simulink library "multiSpoolingController_ul"  (R2020a)
settings: Solver=VariableStepAuto  StartTime=0.0  StopTime=10.0  RelTol=1e-3
undefined symbols (not defined in the file or in its folder): pathCtrl
libraries: firstOrderFilter_ul x1
settings Model: Creator=James Reed  LastModifiedBy=Josh Gaming
settings DataIOCC: ReturnWorkspaceOutputs=off
settings DebuggingCC: ArithmeticOperatorsInVariantConditions=warning
settings SFSimCC: CustomCodeUndefinedFunction=UseInterfaceOnly

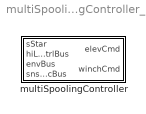
== system multiSpoolingController_ul ==
  multiSpoolingController : Subsystem

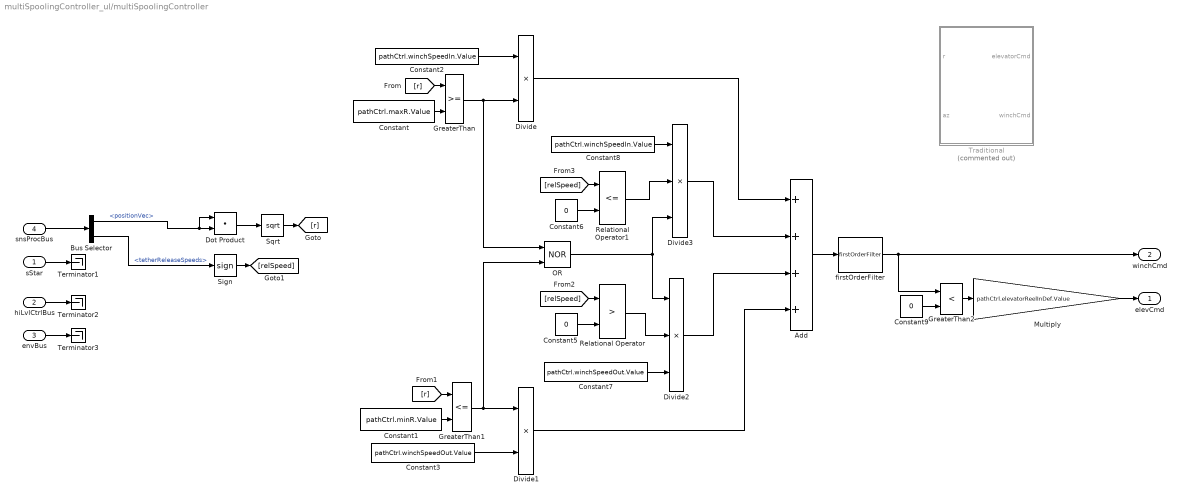
== system multiSpoolingController_ul/multiSpoolingController ==
  "sStar " : Inport
  hiLvlCtrlBus : Inport  Port=2  OutDataTypeStr=Bus: hiLvlCtrlBus
  envBus : Inport  Port=3  OutDataTypeStr=Bus: envBus
  snsProcBus : Inport  Port=4  OutDataTypeStr=Bus: sensorsProcessingBus
  Add : Sum  Inputs=++++
  Bus Selector : BusSelector  OutputSignals=positionVec,tetherReleaseSpeeds
  Constant : Constant  Value=pathCtrl.maxR.Value
  Constant1 : Constant  Value=pathCtrl.minR.Value
  Constant2 : Constant  Value=pathCtrl.winchSpeedIn.Value
  Constant3 : Constant  Value=pathCtrl.winchSpeedOut.Value
  Constant5 : Constant  Value=0
  Constant6 : Constant  Value=0
  Constant7 : Constant  Value=pathCtrl.winchSpeedOut.Value
  Constant8 : Constant  Value=pathCtrl.winchSpeedIn.Value
  Constant9 : Constant  Value=0
  Divide : Product  Inputs=**  OutDataTypeStr=double
  Divide1 : Product  Inputs=**  OutDataTypeStr=double
  Divide2 : Product  Inputs=***  OutDataTypeStr=double
  Divide3 : Product  Inputs=***  OutDataTypeStr=double
  Dot Product : DotProduct  InputSameDT=on  OutDataTypeStr=Inherit: Inherit via internal rule
  GreaterThan : RelationalOperator  OutDataTypeStr=boolean  RndMeth=Simplest
  GreaterThan1 : RelationalOperator  Operator=<=  OutDataTypeStr=boolean  RndMeth=Simplest
  GreaterThan2 : RelationalOperator  Operator=<  OutDataTypeStr=boolean  RndMeth=Simplest
  Multiply : Gain  Gain=pathCtrl.elevatorReelInDef.Value  OutDataTypeStr=double
  OR : Logic  Operator=NOR  AllPortsSameDT=off  OutDataTypeStr=boolean
  Relational Operator : RelationalOperator  Operator=>  OutDataTypeStr=boolean  RndMeth=Simplest
  Relational Operator1 : RelationalOperator  Operator=<=  OutDataTypeStr=boolean  RndMeth=Simplest
  Sign : Signum
  Sqrt : Sqrt  SaturateOnIntegerOverflow=on
  Terminator1 : Terminator
  Terminator2 : Terminator
  Terminator3 : Terminator
  Traditional : Stateflow chart  Commented=on  TreatAsAtomicUnit=on  mask{maxR=pathCtrl.maxR.Value, minR=pathCtrl.minR.Value, winchSpeedIn=pathCtrl.winchSpeedIn.Value, winchSpeedOut=pathCtrl.winchSpeedOut.Value, elevatorReelInDef=pathCtrl.elevatorReelInDef.Value}
      mask prompts: maxR "Min tether length"; minR "Max tether length"; winchSpeedIn "Spool in speed"; winchSpeedOut "Spool out speed"; elevatorReelInDef "Elevator deflection during spool in"
  firstOrderFilter : firstOrderFilter_ul/firstOrderFilter  tau=1  ic=0
  elevCmd : Outport  VectorParamsAs1DForOutWhenUnconnected=off
  "winchCmd " : Outport  Port=2  VectorParamsAs1DForOutWhenUnconnected=off
  wires:
  Multiply/1 -> elevCmd/1
  Add/1 -> firstOrderFilter/1
  firstOrderFilter/1 -> GreaterThan2/1, "winchCmd "/1
  Bus Selector/1 -> Dot Product/2, Dot Product/1  "<positionVec>"
  "sStar "/1 -> Terminator1/1
  Sqrt/1 -> [r]
  Dot Product/1 -> Sqrt/1
  snsProcBus/1 -> Bus Selector/1
  hiLvlCtrlBus/1 -> Terminator2/1
  envBus/1 -> Terminator3/1
  Bus Selector/2 -> Sign/1  "<tetherReleaseSpeeds>"
  Sign/1 -> [relSpeed]
  [r] -> GreaterThan/1
  Constant/1 -> GreaterThan/2
  GreaterThan/1 -> OR/1, Divide/2
  Constant2/1 -> Divide/1
  Constant1/1 -> GreaterThan1/2
  [r] -> GreaterThan1/1
  GreaterThan1/1 -> OR/2, Divide1/1
  Constant3/1 -> Divide1/2
  [relSpeed] -> Relational Operator/1
  Divide/1 -> Add/1
  Constant5/1 -> Relational Operator/2
  Relational Operator/1 -> Divide2/2
  OR/1 -> Divide3/3, Divide2/1
  [relSpeed] -> Relational Operator1/1
  Relational Operator1/1 -> Divide3/2
  Constant6/1 -> Relational Operator1/2
  Constant7/1 -> Divide2/3
  Constant8/1 -> Divide3/1
  Divide3/1 -> Add/2
  Divide2/1 -> Add/3
  Divide1/1 -> Add/4
  Constant9/1 -> GreaterThan2/2
  GreaterThan2/1 -> Multiply/1

== stateflow chart multiSpoolingController_ul/multiSpoolingController/Traditional ==
  state SpoolOut
    entry:
    winchCmd = winchSpeedOut;
    elevatorCmd = 0;
  state SpoolIn
    winchCmd = winchSpeedIn;
    elevatorCmd = elevatorReelInDef;
  (default) -> SpoolIn
  SpoolOut -> SpoolIn : [r > maxR ]
  SpoolIn -> SpoolOut : [r < minR]
  data: elevatorCmd output; r input; az input; winchCmd output; elevatorReelInDef parameter; winchSpeedOut parameter; winchSpeedIn parameter; minR parameter; maxR parameter
